simulink model "PWM2010a_analysis"  (Simulink 7.9)
settings: Solver=ode23tb  StartTime=0.0  StopTime=1.5  FixedStep=0.00001  RelTol=1e-3
libraries: powerlib x15, powerlib_extras x4, simulink x1
settings Model: Creator=zhou  LastModifiedBy=H002220
settings OptimizationCC: InitFltsAndDblsToZero=on
settings DebuggingCC: SaveWithParameterizedLinksMsg=none  SignalResolutionControl=TryResolveAllWithWarning  MultiTaskDSMMsg=warning  MultiTaskCondExecSysMsg=none  FcnCallInpInsideContextMsg=Use local settings
settings CodeAppCC: CustomSymbolStrType=$N$R$M_T
settings GRTTargetCC: TargetFcnLib=ansi_tfl_tmw.mat  CodeReplacementLibrary=C89/C90 (ANSI)  CombineOutputUpdateFcns=off  GRTInterface=on

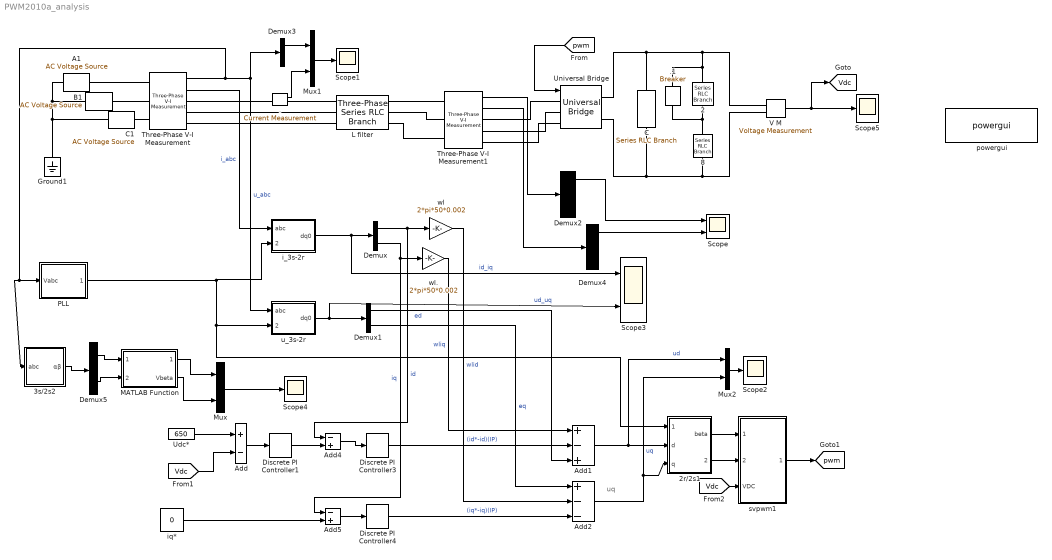
== system PWM2010a_analysis ==
  note: uq
  . : powerlib/Measurements/Current Measurement  PhasorSimulation=off  OutputType=Complex  PSBequivalent=0
  .1 : powerlib/Elements/Breaker  BreakerResistance=0.001  InitialState=0  SnubberResistance=1e6  SnubberCapacitance=inf  SwitchingTimes=[2]  External=off  Measurements=None  MoreParameters=off  NoBreakLoop=off
      settings: AttributesFormatString=\n
  2 : powerlib/Elements/Series RLC Branch  LConnTagsString=__new0  RConnTagsString=__new0  BranchType=R  Resistance=2  Inductance=1e-3  SetiL0=off  InitialCurrent=0  Capacitance=1e-3  Setx0=off  InitialVoltage=0  Measurements=None
  2r/2s1 : Subsystem
  3s/2s2 : Subsystem
  8 : powerlib/Elements/Series RLC Branch  LConnTagsString=__new0  RConnTagsString=__new0  BranchType=R  Resistance=8  Inductance=1e-3  SetiL0=off  InitialCurrent=0  Capacitance=1e-3  Setx0=off  InitialVoltage=0  Measurements=None
  A1 : powerlib/Electrical Sources/AC Voltage Source  Amplitude=311  Phase=90  Frequency=50  SampleTime=0  Measurements=None
  Add : Sum  Inputs=+-
  Add1 : Sum  Inputs=+-+
  Add2 : Sum  Inputs=+--
  Add4 : Sum  Inputs=-+
  Add5 : Sum  Inputs=-+
  B1 : powerlib/Electrical Sources/AC Voltage Source  Amplitude=311  Phase=-120+90  Frequency=50  SampleTime=0  Measurements=None
  "C " : powerlib/Elements/Series RLC Branch  LConnTagsString=__new0  RConnTagsString=__new0  BranchType=C  Resistance=1  Inductance=1e-3  SetiL0=off  InitialCurrent=0  Capacitance=0.008  Setx0=off  InitialVoltage=600  Measurements=None
  C1 : powerlib/Electrical Sources/AC Voltage Source  Amplitude=311  Phase=-240+90  Frequency=50  SampleTime=0  Measurements=None
  Demux : Demux  Outputs=2
  Demux1 : Demux  Outputs=2
  Demux2 : Demux  Outputs=3
  Demux3 : Demux  Outputs=3
  Demux4 : Demux  Outputs=3
  Demux5 : Demux  Outputs=2
  Discrete PI Controller1 : powerlib_extras/Discrete  Control Blocks/Discrete PI Controller  Kp=0.5  Ki=13  Par_Limits=[10000 -10000]  Init=0  Ts=50e-6
  Discrete PI Controller3 : powerlib_extras/Discrete  Control Blocks/Discrete PI Controller  Kp=20  Ki=120  Par_Limits=[1e6 -1e6]  Init=0  Ts=50e-6
  Discrete PI Controller4 : powerlib_extras/Discrete  Control Blocks/Discrete PI Controller  Kp=20  Ki=100  Par_Limits=[1e6 -1e6]  Init=0  Ts=50e-6
  Ground1 : powerlib/Elements/Ground  LConnTagsString=a
  L filter : powerlib/Elements/Three-Phase Series RLC Branch  LConnTagsString=A|B|C  RConnTagsString=A|B|C  BranchType=RL  Resistance=0.5  Inductance=0.002  Capacitance=1e-6  Measurements=None
  MATLAB Function : MATLAB Function  TreatAsAtomicUnit=on
  Mux : Mux  Inputs=2
  Mux1 : Mux  Inputs=2
  Mux2 : Mux  Inputs=2
  PLL : Subsystem
  Scope : Scope  NumInputPorts=2
      settings: YMin=-5~-5  YMax=5~5
  Scope{1..2,4..5} (4 alike) : Scope
      Scope1 settings: YMin=-479.93424  YMax=406.4876
      Scope2 settings: YMin=-7003.21346  YMax=2298.48553  SaveName=ScopeData2
      Scope4 settings: SaveName=ScopeData4
      Scope5 settings: YMin=461.71177  YMax=790.31086  SaveName=ScopeData5
  Scope3 : Scope  NumInputPorts=2
      settings: YMin=-344.98603~-44.36843  YMax=420.48098~350.48538  SaveName=ScopeData3
  Three-Phase V-I Measurement : powerlib/Measurements/Three-Phase V-I Measurement  VoltageMeasurement=phase-to-ground  SetLabelV=off  LabelV=Vabc  Vpu=off  VpuLL=off  CurrentMeasurement=yes  SetLabelI=off  LabelI=Iabc  Ipu=off  Pbase=100e6  Vbase=500e3  OutputType=Complex  PhasorSimulation=off  PSBequivalent=0
  Three-Phase V-I Measurement1 : powerlib/Measurements/Three-Phase V-I Measurement  VoltageMeasurement=phase-to-phase  SetLabelV=off  LabelV=Vabc  Vpu=off  VpuLL=off  CurrentMeasurement=yes  SetLabelI=off  LabelI=Iabc  Ipu=off  Pbase=100e6  Vbase=500e3  OutputType=Complex  PhasorSimulation=off  PSBequivalent=0
  Udc* : Constant  Value=650
  Universal Bridge : powerlib/Power Electronics/Universal Bridge  Arms=3  SnubberResistance=1e5  SnubberCapacitance=inf  Device=IGBT / Diodes  Ron=1e-3  Lon=0  ForwardVoltages="[  0  0  ]"  ForwardVoltage=0  GTOparameters=[ 10e-6 , 20e-6 ]  IGBTparameters=[ 1e-6 , 2e-6 ]  Measurements=None  Measurements_2=None  converterType=Rectifier
  V M : powerlib/Measurements/Voltage Measurement  PhasorSimulation=off  OutputType=Complex  PSBequivalent=0
  i_3s-2r : Subsystem  AncestorBlock=powerlib_extras/Measurements/abc_to_dq0 Transformation
      mask Type: abc to dq0 Transformation
      mask Description:
      | This block performs the  abc to dq0 transformation on a set of three-phase signals. It computes the direct axis Vd, quadratic axis Vq, and zero sequence V0 quantities in a two axis rotating reference frame according to the following transformation:
      | 
      | 
      | Vd = 2/3*[Va*cos(wt) + Vb*cos(wt-2pi/3) + Vc*cos(wt+2pi/3)]
      | Vq = 2/3*[-Va*sin(wt) - Vb*sin(wt-2pi/3) - Vc*sin(wt+2pi/3)]
      | V0 = 1/3*[Va +  Vb  +  Vc ]
      | 
      | where w=  rotation speed (rad/s) of the rotating frame.
      | 
      | This transformation is commonly used in three-phase electric machine models where it is known as the Park transformation.
      mask Help: web(psbhelp);
  iq* : Constant  Value=0
  powergui : powerlib/powergui  SimulationMode=Discrete  SolverType=Tustin  SampleTime=50e-6  frequency=60  SPID=off  DisableSnubberDevices=off  DisableRonSwitches=off  DisableVfSwitches=off  SwTol=0  Interpol=off  DisplayEquations=off  FunctionMessages=off  frequencyindice=0  Pbase=100e6  ErrMax=1e-4  Iterations=50  UnitsV=kV  UnitsW=MW  echomessages=off  HookPort=off  EnableUseOfTLC=off  x0status=blocks  RestoreLinks=warning  ResistiveCurrentMeasurement=off  Frange=[0:2:500]  Ylog=off  Xlog=on  ShowGrid=off  save=off  variable=ZData  structure=ScopeData7  ZoomFFT=on  StartTime=0.4  cycles=2  DisplayStyle=1  fundamental=50  FreqAxis=on  MaxFrequency=1000  frequencyindicesteady=1  RmsSteady=1  display=off  Ts=0  methode=off
  svpwm1 : Subsystem
  u_3s-2r : Subsystem  AncestorBlock=powerlib_extras/Measurements/abc_to_dq0 Transformation
      mask Type: abc to dq0 Transformation
      mask Description:
      | This block performs the  abc to dq0 transformation on a set of three-phase signals. It computes the direct axis Vd, quadratic axis Vq, and zero sequence V0 quantities in a two axis rotating reference frame according to the following transformation:
      | 
      | 
      | Vd = 2/3*[Va*cos(wt) + Vb*cos(wt-2pi/3) + Vc*cos(wt+2pi/3)]
      | Vq = 2/3*[-Va*sin(wt) - Vb*sin(wt-2pi/3) - Vc*sin(wt+2pi/3)]
      | V0 = 1/3*[Va +  Vb  +  Vc ]
      | 
      | where w=  rotation speed (rad/s) of the rotating frame.
      | 
      | This transformation is commonly used in three-phase electric machine models where it is known as the Park transformation.
      mask Help: web(psbhelp);
  wl : Gain  Gain=2*pi*50*0.002
  wl. : Gain  Gain=2*pi*50*0.002
  tag scope: Vdc=global, pwm=global
  wires:
  Three-Phase V-I Measurement/2 -> i_3s-2r/1(abc)  "i_abc"
  i_3s-2r/1(dq0) -> Demux/1, Scope3/1  "id_iq"
  V M/1 -> Scope5/1, [Vdc]
  Add/1 -> Discrete PI Controller1/1
  Discrete PI Controller1/1 -> Add4/2
  Add4/1 -> Discrete PI Controller3/1
  iq*/1 -> Add5/2
  Add5/1 -> Discrete PI Controller4/1
  Add1/1 -> Mux2/1, 2r/2s1/2(d)  "ud"
  Add2/1 -> Mux2/2, 2r/2s1/3(q)  "uq"
  Discrete PI Controller4/1 -> Add2/3  "(iq*-iq)(IP)"
  Demux/1 -> wl/1, Add4/1  "id"
  Demux/2 -> wl./1, Add5/1  "iq"
  wl/1 -> Add2/2  "wlid"
  Discrete PI Controller3/1 -> Add1/2  "(id*-id)(IP)"
  wl./1 -> Add1/1  "wliq"
  Mux2/1 -> Scope2/1
  Three-Phase V-I Measurement/1 -> u_3s-2r/1(abc), Demux3/1, PLL/1(Vabc), 3s/2s2/1(abc)  "u_abc"
  Mux1/1 -> Scope1/1
  2r/2s1/2(alpha) -> svpwm1/2(usaref)
  2r/2s1/1(beta) -> svpwm1/1(usbref)
  u_3s-2r/1(dq0) -> Demux1/1, Scope3/2  "ud_uq"
  Demux3/1 -> Mux1/1
  ./1 -> Mux1/2
  Demux1/1 -> Add1/3  "ed"
  Demux1/2 -> Add2/1  "eq"
  svpwm1/1(6pulse) -> [pwm]
  [pwm] -> Universal Bridge/1
  Udc*/1 -> Add/1
  [Vdc] -> Add/2
  [Vdc] -> svpwm1/3(VDC)
  PLL/1(sin_cos) -> i_3s-2r/2(sin_cos), 2r/2s1/1(sin_cos), u_3s-2r/2(sin_cos)
  Three-Phase V-I Measurement1/1 -> Demux2/1
  Three-Phase V-I Measurement1/2 -> Demux4/1
  Demux4/1 -> Scope/2
  Demux2/1 -> Scope/1
  3s/2s2/1(αβ) -> Demux5/1
  Demux5/2 -> MATLAB Function/2(VbetaL)
  Demux5/1 -> MATLAB Function/1(ValphaL)
  MATLAB Function/1(Valpha) -> Mux/1
  MATLAB Function/2(Vbeta) -> Mux/2
  Mux/1 -> Scope4/1
  connections:
  B1/RConn1 -- Three-Phase V-I Measurement/LConn2
  C1/RConn1 -- Three-Phase V-I Measurement/LConn3
  Three-Phase V-I Measurement/RConn1 -- ./LConn1
  ./RConn1 -- L filter/LConn1
  Ground1/LConn1 -- C1/LConn1 -- A1/LConn1 -- B1/LConn1
  A1/RConn1 -- Three-Phase V-I Measurement/LConn1
  2/RConn1 -- 8/LConn1 -- .1/RConn1
  Three-Phase V-I Measurement/RConn2 -- L filter/LConn2
  Three-Phase V-I Measurement/RConn3 -- L filter/LConn3
  "C "/RConn1 -- 8/RConn1 -- V M/LConn2 -- Universal Bridge/RConn2
  "C "/LConn1 -- Universal Bridge/RConn1 -- 2/LConn1 -- .1/LConn1 -- V M/LConn1
  Three-Phase V-I Measurement1/LConn1 -- L filter/RConn1
  Three-Phase V-I Measurement1/LConn2 -- L filter/RConn2
  Three-Phase V-I Measurement1/LConn3 -- L filter/RConn3
  Three-Phase V-I Measurement1/RConn1 -- Universal Bridge/LConn1
  Three-Phase V-I Measurement1/RConn2 -- Universal Bridge/LConn2
  Three-Phase V-I Measurement1/RConn3 -- Universal Bridge/LConn3

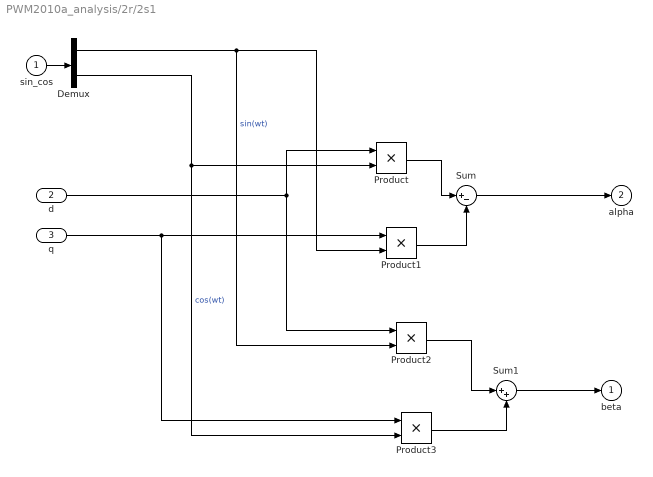
== system PWM2010a_analysis/2r/2s1 ==
  sin_cos : Inport  PortDimensions=2
  d : Inport  Port=2
  q : Inport  Port=3
  Demux : Demux  Outputs=2
  Product{,1..3} (4 alike) : Product  RndMeth=Zero
  Sum : Sum  Inputs=|+-
  Sum1 : Sum  Inputs=|++
  beta : Outport  InitialOutput=0
  alpha : Outport  Port=2  InitialOutput=0
  wires:
  Sum/1 -> alpha/1
  Demux/1 -> Product1/2, Product2/2  "sin(wt)"
  Demux/2 -> Product/2, Product3/2  "cos(wt)"
  sin_cos/1 -> Demux/1
  d/1 -> Product/1, Product2/1
  q/1 -> Product1/1, Product3/1
  Product/1 -> Sum/1
  Product1/1 -> Sum/2
  Product2/1 -> Sum1/1
  Product3/1 -> Sum1/2
  Sum1/1 -> beta/1

== system PWM2010a_analysis/3s/2s2 ==
  abc : Inport
  Demux : Demux  Outputs=3
  MATLAB Function : MATLAB Function  TreatAsAtomicUnit=on
  Mux : Mux  Inputs=2
  αβ : Outport
  wires:
  abc/1 -> Demux/1
  Mux/1 -> αβ/1
  Demux/1 -> MATLAB Function/1(Va)
  Demux/2 -> MATLAB Function/2(Vb)
  Demux/3 -> MATLAB Function/3(Vc)
  MATLAB Function/1(Valpha) -> Mux/1
  MATLAB Function/2(Vbeta) -> Mux/2

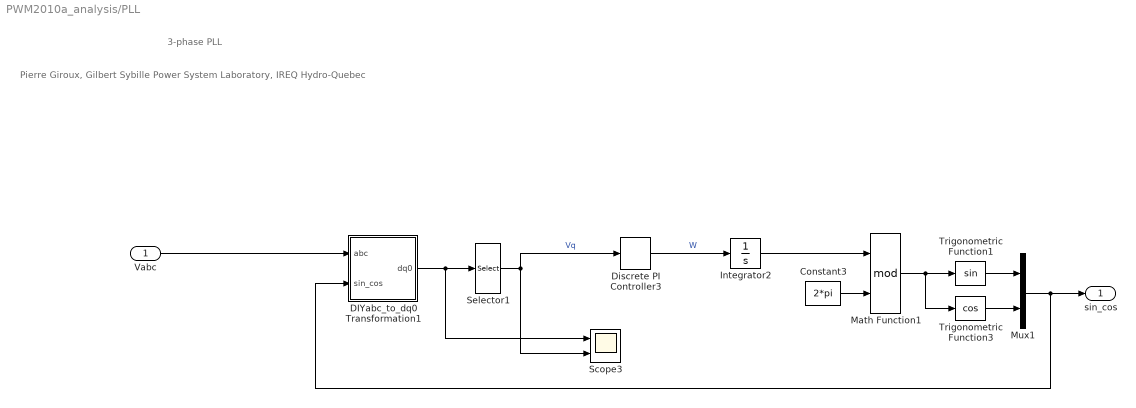
== system PWM2010a_analysis/PLL ==
  note: 3-phase PLL
  note: Pierre Giroux, Gilbert Sybille
      | Power System Laboratory, IREQ
      | Hydro-Quebec
  Vabc : Inport  PortDimensions=3
  Constant3 : Constant  Value=2*pi
  DIYabc_to_dq0 Transformation1 : Subsystem  AncestorBlock=powerlib_extras/Measurements/abc_to_dq0 Transformation
      mask Type: abc to dq0 Transformation
      mask Description:
      | This block performs the  abc to dq0 transformation on a set of three-phase signals. It computes the direct axis Vd, quadratic axis Vq, and zero sequence V0 quantities in a two axis rotating reference frame according to the following transformation:
      | 
      | 
      | Vd = 2/3*[Va*cos(wt) + Vb*cos(wt-2pi/3) + Vc*cos(wt+2pi/3)]
      | Vq = 2/3*[-Va*sin(wt) - Vb*sin(wt-2pi/3) - Vc*sin(wt+2pi/3)]
      | V0 = 1/3*[Va +  Vb  +  Vc ]
      | 
      | where w=  rotation speed (rad/s) of the rotating frame.
      | 
      | This transformation is commonly used in three-phase electric machine models where it is known as the Park transformation.
      mask Help: web(psbhelp);
  Discrete PI Controller3 : powerlib_extras/Discrete  Control Blocks/Discrete PI Controller  Kp=20  Ki=120  Par_Limits=[1e6 -1e6]  Init=0  Ts=50e-6
  Integrator2 : Integrator
  Math Function1 : Math  Operator=mod  SaturateOnIntegerOverflow=on
  Mux1 : Mux  Inputs=2
  Scope3 : Scope  NumInputPorts=2
      settings: YMin=-44.36843~-7.44785  YMax=350.48538~18.20012  SaveName=ScopeData12
  Selector1 : Selector  InputPortWidth=3  IndexOptions=Index vector (dialog)  Indices=2  OutputSizes=1
  Trigonometric Function1 : Trigonometry
  Trigonometric Function3 : Trigonometry  Operator=cos
  sin_cos : Outport
  wires:
  Vabc/1 -> DIYabc_to_dq0 Transformation1/1(abc)
  DIYabc_to_dq0 Transformation1/1(dq0) -> Selector1/1, Scope3/1
  Constant3/1 -> Math Function1/2
  Math Function1/1 -> Trigonometric Function1/1, Trigonometric Function3/1
  Trigonometric Function1/1 -> Mux1/1
  Trigonometric Function3/1 -> Mux1/2
  Mux1/1 -> sin_cos/1, DIYabc_to_dq0 Transformation1/2(sin_cos)
  Discrete PI Controller3/1 -> Integrator2/1  "W"
  Selector1/1 -> Scope3/2, Discrete PI Controller3/1  "Vq"
  Integrator2/1 -> Math Function1/1

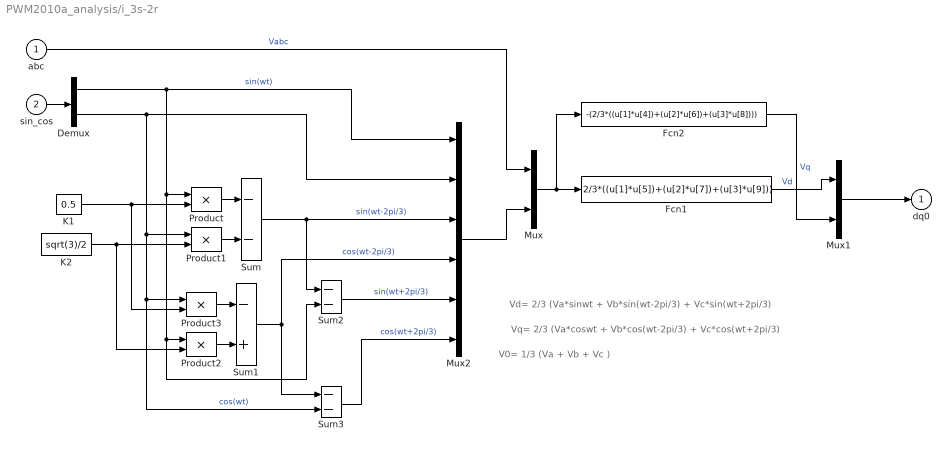
== system PWM2010a_analysis/i_3s-2r ==
  note: V0= 1/3 (Va + Vb + Vc )
  note: Vd= 2/3 (Va*sinwt + Vb*sin(wt-2pi/3) + Vc*sin(wt+2pi/3)
  note: Vq= 2/3 (Va*coswt + Vb*cos(wt-2pi/3) + Vc*cos(wt+2pi/3)
  abc : Inport  PortDimensions=3
  sin_cos : Inport  Port=2  PortDimensions=2
  Demux : Demux  Outputs=2
  Fcn1 : Fcn  Expr=2/3*((u[1]*u[5])+(u[2]*u[7])+(u[3]*u[9]))
  Fcn2 : Fcn  Expr=-(2/3*((u[1]*u[4])+(u[2]*u[6])+(u[3]*u[8])))
  K1 : Constant  Value=0.5
  K2 : Constant  Value=sqrt(3)/2
  Mux : Mux  Inputs=2
  Mux1 : Mux  Inputs=2
  Mux2 : Mux  Inputs=6
  Product{,1..3} (4 alike) : Product  SaturateOnIntegerOverflow=on  InputSameDT=on  OutDataTypeStr=Inherit: Same as first input
  Sum : Sum  Inputs=--  SaturateOnIntegerOverflow=on  InputSameDT=on  OutDataTypeStr=Inherit: Same as first input
  Sum1 : Sum  Inputs=-+  SaturateOnIntegerOverflow=on  InputSameDT=on  OutDataTypeStr=Inherit: Same as first input
  Sum2 : Sum  Inputs=--  SaturateOnIntegerOverflow=on  InputSameDT=on  OutDataTypeStr=Inherit: Same as first input
  Sum3 : Sum  Inputs=--  SaturateOnIntegerOverflow=on  InputSameDT=on  OutDataTypeStr=Inherit: Same as first input
  dq0 : Outport  InitialOutput=0
  wires:
  Fcn1/1 -> Mux1/1  "Vd"
  Fcn2/1 -> Mux1/2  "Vq"
  Mux1/1 -> dq0/1
  Mux/1 -> Fcn1/1, Fcn2/1
  Sum1/1 -> Sum3/1, Mux2/4  "cos(wt-2pi/3)"
  Sum/1 -> Sum2/1, Mux2/3  "sin(wt-2pi/3)"
  K2/1 -> Product2/2, Product1/2
  K1/1 -> Product3/2, Product/2
  Sum2/1 -> Mux2/5  "sin(wt+2pi/3)"
  Sum3/1 -> Mux2/6  "cos(wt+2pi/3)"
  Product2/1 -> Sum1/2
  Product3/1 -> Sum1/1
  Product1/1 -> Sum/2
  Product/1 -> Sum/1
  Demux/1 -> Mux2/1, Sum2/2, Product2/1, Product/1  "sin(wt)"
  Demux/2 -> Mux2/2, Product1/1, Product3/1, Sum3/2  "cos(wt)"
  sin_cos/1 -> Demux/1
  Mux2/1 -> Mux/2
  abc/1 -> Mux/1  "Vabc"

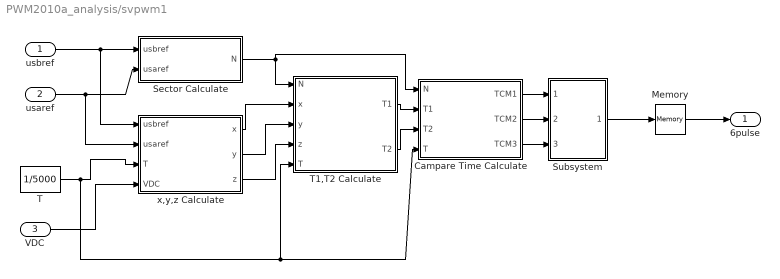
== system PWM2010a_analysis/svpwm1 ==
  usbref : Inport
  usaref : Inport  Port=2
  VDC : Inport  Port=3
  Campare Time Calculate : Subsystem
  Memory : Memory
  Sector Calculate : Subsystem
  Subsystem : Subsystem
  T : Constant  Value=1/5000
  T1,T2 Calculate : Subsystem
  x,y,z Calculate : Subsystem
  6pulse : Outport
  wires:
  usbref/1 -> Sector Calculate/1(usbref), x,y,z Calculate/1(usbref)
  usaref/1 -> Sector Calculate/2(usaref), x,y,z Calculate/2(usaref)
  Sector Calculate/1(N) -> T1,T2 Calculate/1(N), Campare Time Calculate/1(N)
  x,y,z Calculate/1(x) -> T1,T2 Calculate/2(x)
  x,y,z Calculate/2(y) -> T1,T2 Calculate/3(y)
  x,y,z Calculate/3(z) -> T1,T2 Calculate/4(z)
  T1,T2 Calculate/1(T1) -> Campare Time Calculate/2(T1)
  T1,T2 Calculate/2(T2) -> Campare Time Calculate/3(T2)
  Campare Time Calculate/1(TCM1) -> Subsystem/1(TCM1)
  Campare Time Calculate/2(TCM2) -> Subsystem/2(TCM2)
  Campare Time Calculate/3(TCM3) -> Subsystem/3(TCM3)
  Subsystem/1(Out1) -> Memory/1
  T/1 -> x,y,z Calculate/3(T), T1,T2 Calculate/5(T), Campare Time Calculate/4(T)
  VDC/1 -> x,y,z Calculate/4(VDC)
  Memory/1 -> 6pulse/1

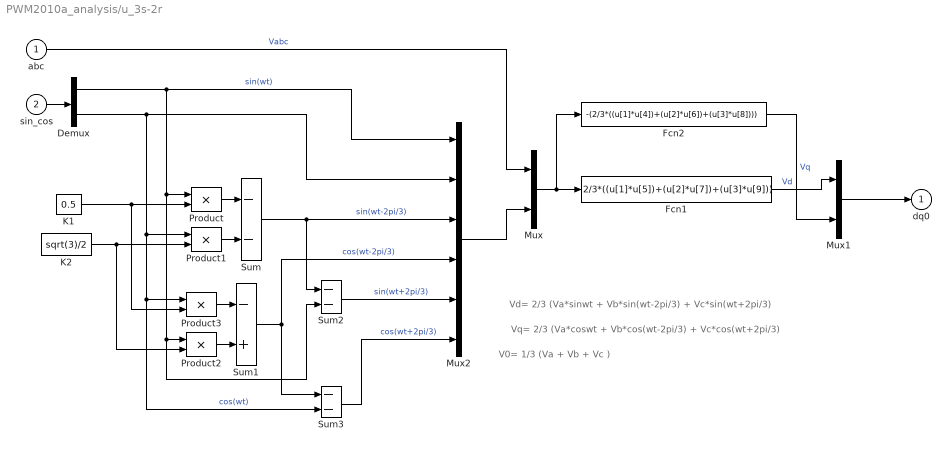
== system PWM2010a_analysis/u_3s-2r ==
  note: Vq= 2/3 (Va*coswt + Vb*cos(wt-2pi/3) + Vc*cos(wt+2pi/3)
  note: Vd= 2/3 (Va*sinwt + Vb*sin(wt-2pi/3) + Vc*sin(wt+2pi/3)
  note: V0= 1/3 (Va + Vb + Vc )
  abc : Inport  PortDimensions=3
  sin_cos : Inport  Port=2  PortDimensions=2
  Demux : Demux  Outputs=2
  Fcn1 : Fcn  Expr=2/3*((u[1]*u[5])+(u[2]*u[7])+(u[3]*u[9]))
  Fcn2 : Fcn  Expr=-(2/3*((u[1]*u[4])+(u[2]*u[6])+(u[3]*u[8])))
  K1 : Constant  Value=0.5
  K2 : Constant  Value=sqrt(3)/2
  Mux : Mux  Inputs=2
  Mux1 : Mux  Inputs=2
  Mux2 : Mux  Inputs=6
  Product{,1..3} (4 alike) : Product  SaturateOnIntegerOverflow=on  InputSameDT=on  OutDataTypeStr=Inherit: Same as first input
  Sum : Sum  Inputs=--  SaturateOnIntegerOverflow=on  InputSameDT=on  OutDataTypeStr=Inherit: Same as first input
  Sum1 : Sum  Inputs=-+  SaturateOnIntegerOverflow=on  InputSameDT=on  OutDataTypeStr=Inherit: Same as first input
  Sum2 : Sum  Inputs=--  SaturateOnIntegerOverflow=on  InputSameDT=on  OutDataTypeStr=Inherit: Same as first input
  Sum3 : Sum  Inputs=--  SaturateOnIntegerOverflow=on  InputSameDT=on  OutDataTypeStr=Inherit: Same as first input
  dq0 : Outport  InitialOutput=0
  wires:
  abc/1 -> Mux/1  "Vabc"
  Mux2/1 -> Mux/2
  sin_cos/1 -> Demux/1
  Demux/2 -> Sum3/2, Product3/1, Product1/1, Mux2/2  "cos(wt)"
  Demux/1 -> Product/1, Product2/1, Sum2/2, Mux2/1  "sin(wt)"
  Product/1 -> Sum/1
  Product1/1 -> Sum/2
  Product3/1 -> Sum1/1
  Product2/1 -> Sum1/2
  Sum3/1 -> Mux2/6  "cos(wt+2pi/3)"
  Sum2/1 -> Mux2/5  "sin(wt+2pi/3)"
  K1/1 -> Product/2, Product3/2
  K2/1 -> Product1/2, Product2/2
  Sum/1 -> Mux2/3, Sum2/1  "sin(wt-2pi/3)"
  Sum1/1 -> Mux2/4, Sum3/1  "cos(wt-2pi/3)"
  Mux/1 -> Fcn2/1, Fcn1/1
  Mux1/1 -> dq0/1
  Fcn2/1 -> Mux1/2  "Vq"
  Fcn1/1 -> Mux1/1  "Vd"

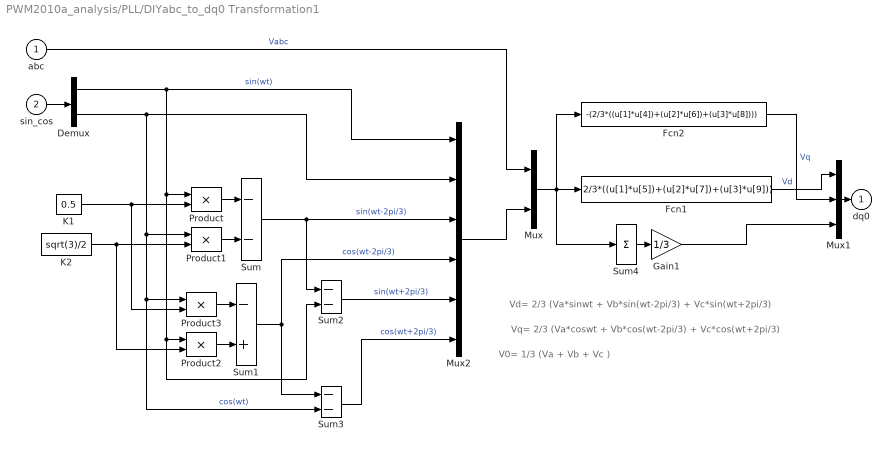
== system PWM2010a_analysis/PLL/DIYabc_to_dq0 Transformation1 ==
  note: V0= 1/3 (Va + Vb + Vc )
  note: Vd= 2/3 (Va*sinwt + Vb*sin(wt-2pi/3) + Vc*sin(wt+2pi/3)
  note: Vq= 2/3 (Va*coswt + Vb*cos(wt-2pi/3) + Vc*cos(wt+2pi/3)
  abc : Inport  PortDimensions=3
  sin_cos : Inport  Port=2  PortDimensions=2
  Demux : Demux  Outputs=2
  Fcn1 : Fcn  Expr=2/3*((u[1]*u[5])+(u[2]*u[7])+(u[3]*u[9]))
  Fcn2 : Fcn  Expr=-(2/3*((u[1]*u[4])+(u[2]*u[6])+(u[3]*u[8])))
  Gain1 : Gain  Gain=1/3  SaturateOnIntegerOverflow=on  OutDataTypeStr=Inherit: Same as input  ParamDataTypeStr=Inherit: Same as input
  K1 : Constant  Value=0.5
  K2 : Constant  Value=sqrt(3)/2
  Mux : Mux  Inputs=2
  Mux1 : Mux  Inputs=3
  Mux2 : Mux  Inputs=6
  Product{,1..3} (4 alike) : Product  SaturateOnIntegerOverflow=on  InputSameDT=on  OutDataTypeStr=Inherit: Same as first input
  Sum : Sum  Inputs=--  SaturateOnIntegerOverflow=on  InputSameDT=on  OutDataTypeStr=Inherit: Same as first input
  Sum1 : Sum  Inputs=-+  SaturateOnIntegerOverflow=on  InputSameDT=on  OutDataTypeStr=Inherit: Same as first input
  Sum2 : Sum  Inputs=--  SaturateOnIntegerOverflow=on  InputSameDT=on  OutDataTypeStr=Inherit: Same as first input
  Sum3 : Sum  Inputs=--  SaturateOnIntegerOverflow=on  InputSameDT=on  OutDataTypeStr=Inherit: Same as first input
  Sum4 : Sum  Inputs=1  SaturateOnIntegerOverflow=on  InputSameDT=on  OutDataTypeStr=Inherit: Same as first input
  dq0 : Outport  InitialOutput=0
  wires:
  Fcn1/1 -> Mux1/1  "Vd"
  Fcn2/1 -> Mux1/2  "Vq"
  Mux1/1 -> dq0/1
  Sum4/1 -> Gain1/1
  Mux/1 -> Sum4/1, Fcn1/1, Fcn2/1
  Sum1/1 -> Sum3/1, Mux2/4  "cos(wt-2pi/3)"
  Sum/1 -> Sum2/1, Mux2/3  "sin(wt-2pi/3)"
  K2/1 -> Product2/2, Product1/2
  K1/1 -> Product3/2, Product/2
  Sum2/1 -> Mux2/5  "sin(wt+2pi/3)"
  Sum3/1 -> Mux2/6  "cos(wt+2pi/3)"
  Product2/1 -> Sum1/2
  Product3/1 -> Sum1/1
  Product1/1 -> Sum/2
  Product/1 -> Sum/1
  Demux/1 -> Mux2/1, Sum2/2, Product2/1, Product/1  "sin(wt)"
  Demux/2 -> Mux2/2, Product1/1, Product3/1, Sum3/2  "cos(wt)"
  sin_cos/1 -> Demux/1
  Mux2/1 -> Mux/2
  abc/1 -> Mux/1  "Vabc"
  Gain1/1 -> Mux1/3

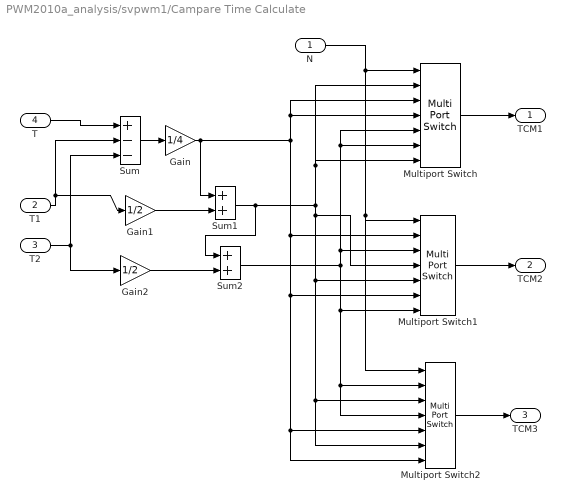
== system PWM2010a_analysis/svpwm1/Campare Time Calculate ==
  N : Inport
  T1 : Inport  Port=2
  T2 : Inport  Port=3
  T : Inport  Port=4
  Gain : Gain  Gain=1/4  SaturateOnIntegerOverflow=on  OutDataTypeStr=Inherit: Same as input  ParamDataTypeStr=Inherit: Same as input
  Gain1 : Gain  Gain=1/2  SaturateOnIntegerOverflow=on  OutDataTypeStr=Inherit: Same as input  ParamDataTypeStr=Inherit: Same as input
  Gain2 : Gain  Gain=1/2  SaturateOnIntegerOverflow=on  OutDataTypeStr=Inherit: Same as input  ParamDataTypeStr=Inherit: Same as input
  Multiport Switch : MultiPortSwitch  Inputs=6  zeroidx=off  SaturateOnIntegerOverflow=on
  Multiport Switch1 : MultiPortSwitch  Inputs=6  zeroidx=off  SaturateOnIntegerOverflow=on
  Multiport Switch2 : MultiPortSwitch  Inputs=6  zeroidx=off  SaturateOnIntegerOverflow=on
  Sum : Sum  Inputs=+--  SaturateOnIntegerOverflow=on
  Sum1 : Sum  SaturateOnIntegerOverflow=on
  Sum2 : Sum  SaturateOnIntegerOverflow=on
  TCM1 : Outport
  TCM2 : Outport  Port=2
  TCM3 : Outport  Port=3
  wires:
  T/1 -> Sum/1
  T1/1 -> Sum/2, Gain1/1
  T2/1 -> Sum/3, Gain2/1
  Sum/1 -> Gain/1
  Gain/1 -> Sum1/1, Multiport Switch1/2, Multiport Switch2/5, Multiport Switch2/7, Multiport Switch1/6, Multiport Switch/3, Multiport Switch/4
  Gain1/1 -> Sum1/2
  Gain2/1 -> Sum2/2
  Multiport Switch1/1 -> TCM2/1
  Multiport Switch/1 -> TCM1/1
  Multiport Switch2/1 -> TCM3/1
  N/1 -> Multiport Switch/1, Multiport Switch2/1, Multiport Switch1/1
  Sum1/1 -> Sum2/1, Multiport Switch1/4, Multiport Switch2/3, Multiport Switch2/6, Multiport Switch1/5, Multiport Switch/2, Multiport Switch/7
  Sum2/1 -> Multiport Switch1/3, Multiport Switch/6, Multiport Switch/5, Multiport Switch2/2, Multiport Switch2/4, Multiport Switch1/7

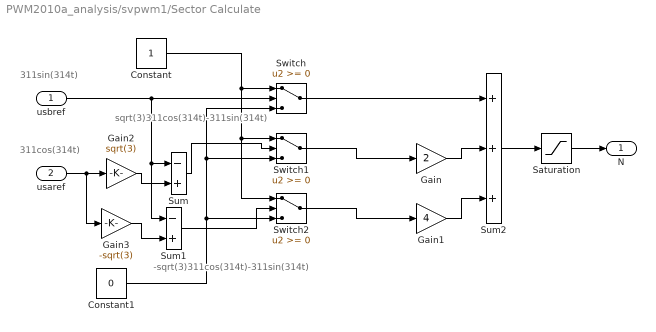
== system PWM2010a_analysis/svpwm1/Sector Calculate ==
  note: 311sin(314t)
  note: 311cos(314t)
  note: sqrt(3)311cos(314t)-311sin(314t)
  note: -sqrt(3)311cos(314t)-311sin(314t)
  usbref : Inport
  usaref : Inport  Port=2
  Constant : Constant
  Constant1 : Constant  Value=0
  Gain : Gain  Gain=2  SaturateOnIntegerOverflow=on  OutDataTypeStr=Inherit: Same as input  ParamDataTypeStr=Inherit: Same as input
  Gain1 : Gain  Gain=4  SaturateOnIntegerOverflow=on  OutDataTypeStr=Inherit: Same as input  ParamDataTypeStr=Inherit: Same as input
  Gain2 : Gain  Gain=sqrt(3)  SaturateOnIntegerOverflow=on  OutDataTypeStr=Inherit: Same as input  ParamDataTypeStr=Inherit: Same as input
  Gain3 : Gain  Gain=-sqrt(3)  SaturateOnIntegerOverflow=on  OutDataTypeStr=Inherit: Same as input  ParamDataTypeStr=Inherit: Same as input
  Saturation : Saturate  UpperLimit=6  LowerLimit=1
  Sum : Sum  Inputs=-+  SaturateOnIntegerOverflow=on
  Sum1 : Sum  Inputs=-+  SaturateOnIntegerOverflow=on
  Sum2 : Sum  Inputs=+++  SaturateOnIntegerOverflow=on
  Switch : Switch  SaturateOnIntegerOverflow=on
  Switch1 : Switch  SaturateOnIntegerOverflow=on
  Switch2 : Switch  SaturateOnIntegerOverflow=on
  N : Outport
  wires:
  Constant/1 -> Switch/1, Switch1/1, Switch2/1
  usbref/1 -> Sum/1, Sum1/1, Switch/2
  Constant1/1 -> Switch/3, Switch1/3, Switch2/3
  usaref/1 -> Gain2/1, Gain3/1
  Gain2/1 -> Sum/2
  Gain3/1 -> Sum1/2
  Sum/1 -> Switch1/2
  Sum1/1 -> Switch2/2
  Switch1/1 -> Gain/1
  Switch/1 -> Sum2/1
  Gain/1 -> Sum2/2
  Gain1/1 -> Sum2/3
  Switch2/1 -> Gain1/1
  Sum2/1 -> Saturation/1
  Saturation/1 -> N/1

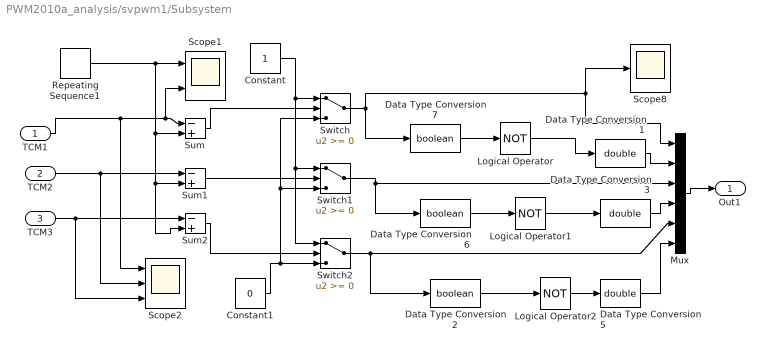
== system PWM2010a_analysis/svpwm1/Subsystem ==
  TCM1 : Inport
  TCM2 : Inport  Port=2
  TCM3 : Inport  Port=3
  Constant : Constant
  Constant1 : Constant  Value=0
  Data Type Conversion1 : DataTypeConversion  OutDataTypeStr=double  SaturateOnIntegerOverflow=on  RndMeth=Zero
  Data Type Conversion2 : DataTypeConversion  OutDataTypeStr=boolean  SaturateOnIntegerOverflow=on  RndMeth=Zero
  Data Type Conversion3 : DataTypeConversion  OutDataTypeStr=double  SaturateOnIntegerOverflow=on  RndMeth=Zero
  Data Type Conversion5 : DataTypeConversion  OutDataTypeStr=double  SaturateOnIntegerOverflow=on  RndMeth=Zero
  Data Type Conversion6 : DataTypeConversion  OutDataTypeStr=boolean  SaturateOnIntegerOverflow=on  RndMeth=Zero
  Data Type Conversion7 : DataTypeConversion  OutDataTypeStr=boolean  SaturateOnIntegerOverflow=on  RndMeth=Zero
  Logical Operator : Logic  Operator=NOT  AllPortsSameDT=off
  Logical Operator1 : Logic  Operator=NOT  AllPortsSameDT=off
  Logical Operator2 : Logic  Operator=NOT  AllPortsSameDT=off
  Mux : Mux  Inputs=6
  Repeating Sequence1 : simulink/Sources/Repeating Sequence  rep_seq_t=[0 1/10000 1/5000]  rep_seq_y=[0 1/10000 0]
  Scope1 : Scope  NumInputPorts=2
      settings: TimeRange=0.028  YMin=0~2.45e-005  YMax=8.5e-005~2.64e-005  SaveName=ScopeData15
  Scope2 : Scope  NumInputPorts=3
      settings: TimeRange=0.07000000000000001  YMin=2.25e-005~2.25e-005~2.25e-005  YMax=6e-005~6e-005~6e-005  SaveName=ScopeData19
  Scope8 : Scope
      settings: TimeRange=0.07000000000000001  YMin=0  YMax=2  SaveName=ScopeData13
  Sum : Sum  Inputs=-+  SaturateOnIntegerOverflow=on
  Sum1 : Sum  Inputs=-+  SaturateOnIntegerOverflow=on
  Sum2 : Sum  Inputs=-+  SaturateOnIntegerOverflow=on
  Switch : Switch  SaturateOnIntegerOverflow=on
  Switch1 : Switch  SaturateOnIntegerOverflow=on
  Switch2 : Switch  SaturateOnIntegerOverflow=on
  Out1 : Outport
  wires:
  Constant/1 -> Switch/1, Switch1/1, Switch2/1
  Constant1/1 -> Switch2/3, Switch/3, Switch1/3
  Repeating Sequence1/1 -> Scope1/1, Sum/2, Sum2/2, Sum1/2
  TCM1/1 -> Sum/1, Scope1/2, Scope2/1
  TCM2/1 -> Sum1/1, Scope2/2
  TCM3/1 -> Sum2/1, Scope2/3
  Sum/1 -> Switch/2
  Sum1/1 -> Switch1/2
  Sum2/1 -> Switch2/2
  Mux/1 -> Out1/1
  Switch/1 -> Scope8/1, Mux/1, Data Type Conversion7/1
  Switch1/1 -> Mux/3, Data Type Conversion6/1
  Switch2/1 -> Data Type Conversion2/1, Mux/5
  Logical Operator2/1 -> Data Type Conversion5/1
  Logical Operator1/1 -> Data Type Conversion3/1
  Logical Operator/1 -> Data Type Conversion1/1
  Data Type Conversion1/1 -> Mux/2
  Data Type Conversion3/1 -> Mux/4
  Data Type Conversion5/1 -> Mux/6
  Data Type Conversion7/1 -> Logical Operator/1
  Data Type Conversion6/1 -> Logical Operator1/1
  Data Type Conversion2/1 -> Logical Operator2/1

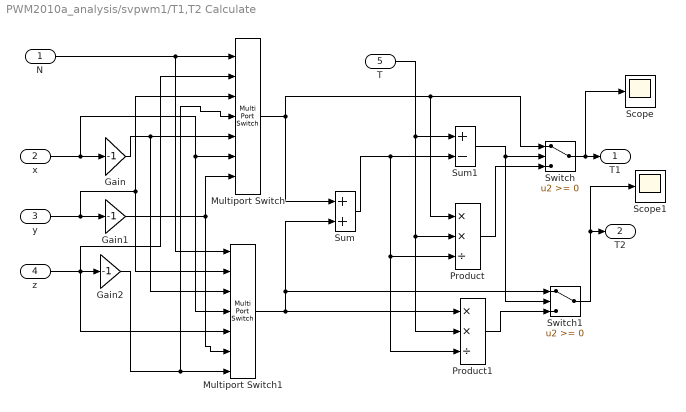
== system PWM2010a_analysis/svpwm1/T1,T2 Calculate ==
  N : Inport
  x : Inport  Port=2
  y : Inport  Port=3
  z : Inport  Port=4
  T : Inport  Port=5
  Gain : Gain  Gain=-1  SaturateOnIntegerOverflow=on  OutDataTypeStr=Inherit: Same as input  ParamDataTypeStr=Inherit: Same as input
  Gain1 : Gain  Gain=-1  SaturateOnIntegerOverflow=on  OutDataTypeStr=Inherit: Same as input  ParamDataTypeStr=Inherit: Same as input
  Gain2 : Gain  Gain=-1  SaturateOnIntegerOverflow=on  OutDataTypeStr=Inherit: Same as input  ParamDataTypeStr=Inherit: Same as input
  Multiport Switch : MultiPortSwitch  Inputs=6  zeroidx=off  SaturateOnIntegerOverflow=on
  Multiport Switch1 : MultiPortSwitch  Inputs=6  zeroidx=off  SaturateOnIntegerOverflow=on
  Product : Product  Inputs=**/  SaturateOnIntegerOverflow=on  OutDataTypeStr=Inherit: Same as first input
  Product1 : Product  Inputs=**/  SaturateOnIntegerOverflow=on  OutDataTypeStr=Inherit: Same as first input
  Scope : Scope
      settings: YMin=3.5e-005  YMax=6.25e-005  SaveName=ScopeData16
  Scope1 : Scope
      settings: YMin=1.3e-007  YMax=2e-007  SaveName=ScopeData17
  Sum : Sum  SaturateOnIntegerOverflow=on
  Sum1 : Sum  Inputs=+-  SaturateOnIntegerOverflow=on
  Switch : Switch  SaturateOnIntegerOverflow=on
  Switch1 : Switch  SaturateOnIntegerOverflow=on
  T1 : Outport
  T2 : Outport  Port=2
  wires:
  N/1 -> Multiport Switch/1, Multiport Switch1/1
  x/1 -> Gain/1, Multiport Switch/6, Multiport Switch1/4
  y/1 -> Gain1/1, Multiport Switch/3, Multiport Switch1/2
  z/1 -> Gain2/1, Multiport Switch1/5, Multiport Switch/2
  Gain/1 -> Multiport Switch/5, Multiport Switch1/3
  Gain1/1 -> Multiport Switch1/6, Multiport Switch/7
  Gain2/1 -> Multiport Switch1/7, Multiport Switch/4
  Multiport Switch/1 -> Sum/1, Switch/1, Product/1
  Multiport Switch1/1 -> Product1/1, Sum/2, Switch1/1
  Switch1/1 -> T2/1, Scope1/1
  Switch/1 -> T1/1, Scope/1
  T/1 -> Sum1/1, Product1/2, Product/2
  Sum/1 -> Sum1/2, Product1/3, Product/3
  Sum1/1 -> Switch/2, Switch1/2
  Product/1 -> Switch/3
  Product1/1 -> Switch1/3

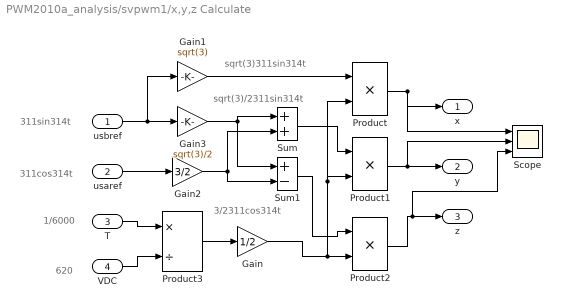
== system PWM2010a_analysis/svpwm1/x,y,z Calculate ==
  note: 311sin314t
  note: 311cos314t
  note: 1/6000
  note: 620
  note: sqrt(3)311sin314t
  note: sqrt(3)/2311sin314t
  note: 3/2311cos314t
  usbref : Inport
  usaref : Inport  Port=2
  T : Inport  Port=3
  VDC : Inport  Port=4
  Gain : Gain  Gain=1/2  SaturateOnIntegerOverflow=on  OutDataTypeStr=Inherit: Same as input  ParamDataTypeStr=Inherit: Same as input
  Gain1 : Gain  Gain=sqrt(3)  SaturateOnIntegerOverflow=on  OutDataTypeStr=Inherit: Same as input  ParamDataTypeStr=Inherit: Same as input
  Gain2 : Gain  Gain=3/2  SaturateOnIntegerOverflow=on  OutDataTypeStr=Inherit: Same as input  ParamDataTypeStr=Inherit: Same as input
  Gain3 : Gain  Gain=sqrt(3)/2  SaturateOnIntegerOverflow=on  OutDataTypeStr=Inherit: Same as input  ParamDataTypeStr=Inherit: Same as input
  Product : Product  SaturateOnIntegerOverflow=on  OutDataTypeStr=Inherit: Same as first input
  Product1 : Product  SaturateOnIntegerOverflow=on  OutDataTypeStr=Inherit: Same as first input
  Product2 : Product  SaturateOnIntegerOverflow=on  OutDataTypeStr=Inherit: Same as first input
  Product3 : Product  Inputs=*/  SaturateOnIntegerOverflow=on  OutDataTypeStr=Inherit: Same as first input
  Scope : Scope  NumInputPorts=3
      settings: YMin=-8e-005~-8e-005~-8e-005  YMax=8e-005~8e-005~8e-005  SaveName=ScopeData18
  Sum : Sum  SaturateOnIntegerOverflow=on
  Sum1 : Sum  Inputs=+-  SaturateOnIntegerOverflow=on
  x : Outport
  y : Outport  Port=2
  z : Outport  Port=3
  wires:
  T/1 -> Product3/1
  VDC/1 -> Product3/2
  usaref/1 -> Gain2/1
  usbref/1 -> Gain3/1, Gain1/1
  Gain1/1 -> Product/1
  Gain/1 -> Product2/2, Product1/2, Product/2
  Gain3/1 -> Sum/1, Sum1/1
  Gain2/1 -> Sum1/2, Sum/2
  Sum/1 -> Product1/1
  Sum1/1 -> Product2/1
  Product/1 -> x/1, Scope/1
  Product1/1 -> y/1, Scope/2
  Product2/1 -> z/1, Scope/3
  Product3/1 -> Gain/1

== matlab function 3s//2s2/MATLAB Function ==
  data: Va input double; Valpha output double; Vb input double; Vc input double; Vbeta output double
function [Valpha, Vbeta] = Park(Va, Vb, Vc)
%#codegen
Valpha = sqrt(2/3)*(Va - Vb/2 -Vc/2);
Vbeta  = sqrt(2/3)*(sqrt(3)*Vb/2 - sqrt(3)*Vc/2);

== matlab function MATLAB Function ==
  data: ValphaL input double; Valpha output double; VbetaL input double; Vbeta output double
function [Valpha, Vbeta] = fcn(ValphaL, VbetaL)
%#将线电压矢量转换成相电压矢量
sin30 = sin(pi/6);
cos30 = cos(pi/6);
Valpha = ( ValphaL*cos30 + VbetaL*sin30)/sqrt(3);
Vbeta  = (-ValphaL*sin30 + VbetaL*cos30)/sqrt(3);
